simulink model "Truth_Table"  (R2021b)
settings: Solver=ode4  StartTime=0.0  StopTime=10.0  FixedStep=10^-5  RelTol=1e-3
settings Model: Creator=t  LastModifiedBy=t

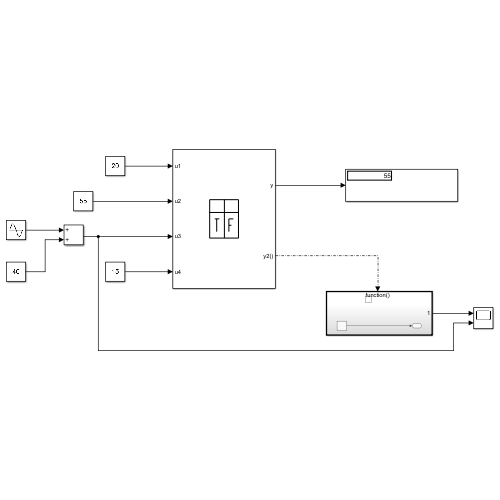
[thumbnail: Simulink's stored preview of the top-level diagram]
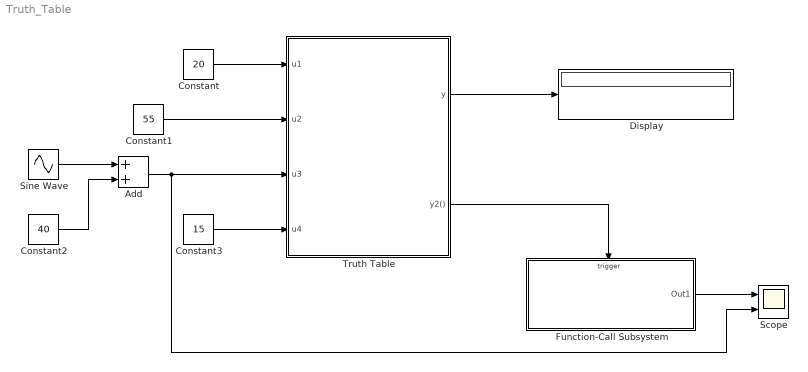
== system Truth_Table ==
  Add : Sum
  Constant : Constant  Value=20
  Constant1 : Constant  Value=55
  Constant2 : Constant  Value=40
  Constant3 : Constant  Value=15
  Display : Display
  Function-Call Subsystem : Subsystem  TreatAsAtomicUnit=on
  Scope : Scope  NumInputPorts=2
  Sine Wave : Sin  Amplitude=40  SampleTime=0
  Truth Table : Truth Table  TreatAsAtomicUnit=on
  wires:
  Constant1/1 -> Truth Table/2(u2)
  Constant/1 -> Truth Table/1(u1)
  Constant3/1 -> Truth Table/4(u4)
  Truth Table/1(y) -> Display/1
  Truth Table/2(y2()) -> Function-Call Subsystem/Trigger
  Function-Call Subsystem/1(Out1) -> Scope/1
  Sine Wave/1 -> Add/1
  Add/1 -> Scope/2, Truth Table/3(u3)
  Constant2/1 -> Add/2

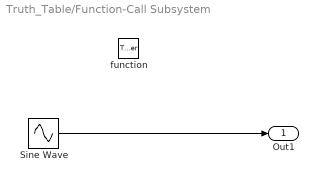
== system Truth_Table/Function-Call Subsystem ==
  function : TriggerPort  TriggerType=function-call  VariantControl=(inherit)
  Sine Wave : Sin
  Out1 : Outport
  wires:
  Sine Wave/1 -> Out1/1

== matlab function Truth_Table/Truth Table ==
  data: u1 input; y output; u2 input; u3 input; u4 input
  events: y2 output FUNCTION_CALL_EVENT
function y = fcn(u1, u2, u3, u4)

aVarTruthTableCondition_1 = false;
aVarTruthTableCondition_2 = false;
aVarTruthTableCondition_3 = false;
aVarTruthTableCondition_4 = false;
aVarTruthTableCondition_5 = false;
aVarTruthTableCondition_6 = false;


% Example condition 1

aVarTruthTableCondition_1 = logical(u1 >u2);

% Example condition 2

aVarTruthTableCondition_2 = logical(u1 >u3);

% Example condition 3

aVarTruthTableCondition_3 = logical(u1 >u4);

% Example condition 4

aVarTruthTableCondition_4 = logical(u2 >u3);

% Example condition 5

aVarTruthTableCondition_5 = logical(u2 >u4);

% Example condition 6

aVarTruthTableCondition_6 = logical(u3 >u4);

if (aVarTruthTableCondition_1 && aVarTruthTableCondition_2 && aVarTruthTableCondition_3)
    aFcnTruthTableAction_1();
elseif (~aVarTruthTableCondition_1 && aVarTruthTableCondition_4 && aVarTruthTableCondition_5)
    aFcnTruthTableAction_2();
elseif (~aVarTruthTableCondition_2 && ~aVarTruthTableCondition_4 && aVarTruthTableCondition_6)
    aFcnTruthTableAction_3();
elseif (~aVarTruthTableCondition_3 && ~aVarTruthTableCondition_5 && ~aVarTruthTableCondition_6)
    aFcnTruthTableAction_4();
else % Default
    aFcnTruthTableAction_1();
end

function aFcnTruthTableAction_1()

% Example action 1 called from D1 & D2 column in condition table

y = u1;

function aFcnTruthTableAction_2()

% Example action 2 called from D3 column in condition table

y = u2;

function aFcnTruthTableAction_3()

% Example action 2 called from D3 column in condition table

y = u3;
y2();

function aFcnTruthTableAction_4()

% Example action 2 called from D3 column in condition table

y = u4;
